simulink model "MBD_If_Action_Subsystem"  (R2021b)
settings: Solver=FixedStepDiscrete  StartTime=0.0  StopTime=10.0  FixedStep=0.001  RelTol=1e-3
libraries: simulink x2
settings Model: Creator=waleed.elshemy  LastModifiedBy=waleed.elshemy
settings OptimizationCC: DefaultParameterBehavior=Inlined  UseDivisionForNetSlopeComputation=on  GainParamInheritBuiltInType=on  UseFloatMulNetSlope=on  InlineInvariantSignals=on  PassReuseOutputArgsAs=Individual arguments  ZeroExternalMemoryAtStartup=off  ZeroInternalMemoryAtStartup=off  NoFixptDivByZeroProtection=on  EfficientFloat2IntCast=on  LifeSpan=1  OptimizeBlockOrder=speed  DifferentSizesBufferReuse=on  EfficientTunableParamExpr=on
settings DebuggingCC: ParameterTunabilityLossMsg=error
settings HardwareCC: ProdLongLongMode=on
settings SFSimCC: MATLABDynamicMemAlloc=off
settings RTWCC: Description=Embedded Coder  SystemTargetFile=ert.tlc  TemplateMakefile=ert_default_tmf
settings CodeAppCC: ForceParamTrailComments=on  IgnoreCustomStorageClasses=off  OperatorAnnotations=on  SimulinkDataObjDesc=on  SFDataObjDesc=on  CustomSymbolStrGlobalVar=rt$N$M  CustomSymbolStrType=$N$M  CustomSymbolStrFcn=$N$M$F  CustomSymbolStrMacro=$N$M  InsertBlockDesc=on
settings ERTTargetCC: TargetLangStandard=C99 (ISO)  GenerateSampleERTMain=on  IncludeMdlTerminateFcn=off  CombineSignalStateStructs=on  SupportComplex=off  SupportContinuousTime=on  InlinedParameterPlacement=NonHierarchical  ERTCustomFileTemplate=example_file_process.tlc  ERTFilePackagingFormat=CompactWithDataFile

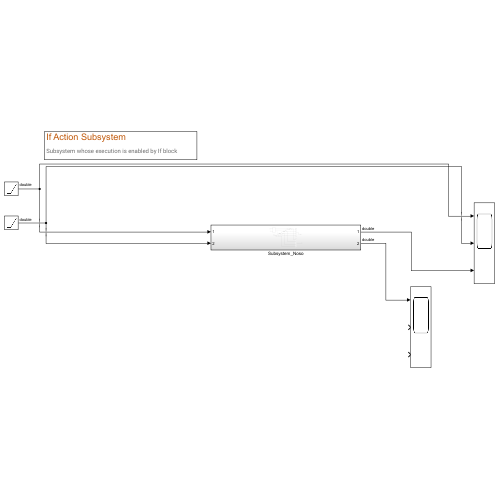
[thumbnail: Simulink's stored preview of the top-level diagram]
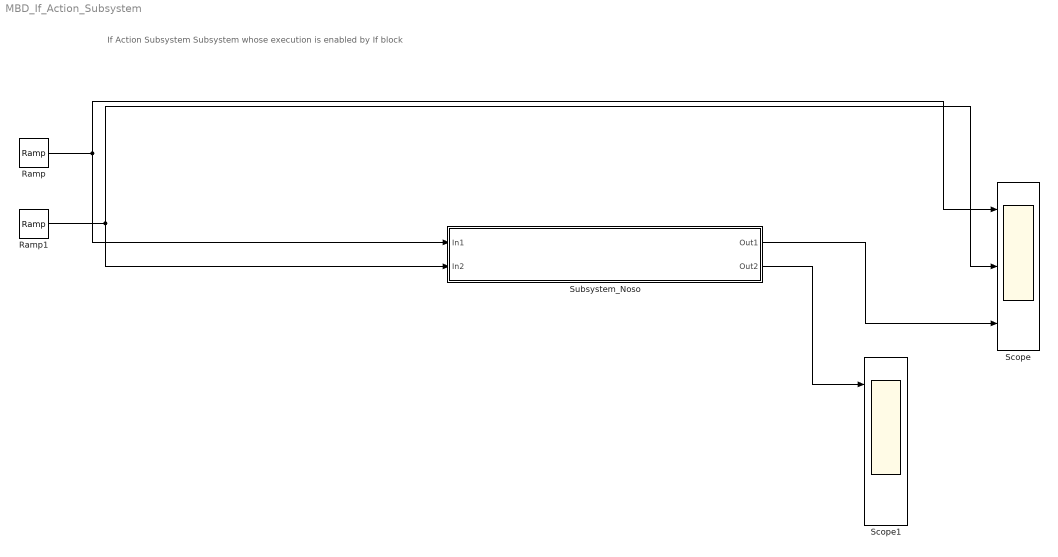
== system MBD_If_Action_Subsystem ==
  note: If Action Subsystem
      | Subsystem whose execution is enabled by If block
  Ramp : simulink/Sources/Ramp  slope=1  start=0  InitialOutput=0
  Ramp1 : simulink/Sources/Ramp  slope=-1  start=0  InitialOutput=10
  Scope : Scope  NumInputPorts=3
  Scope1 : Scope  NumInputPorts=3
  Subsystem_Noso : Subsystem
  wires:
  Ramp/1 -> Subsystem_Noso/1(In1), Scope/1
  Ramp1/1 -> Subsystem_Noso/2(In2), Scope/2
  Subsystem_Noso/1(Out1) -> Scope/3
  Subsystem_Noso/2(Out2) -> Scope1/1

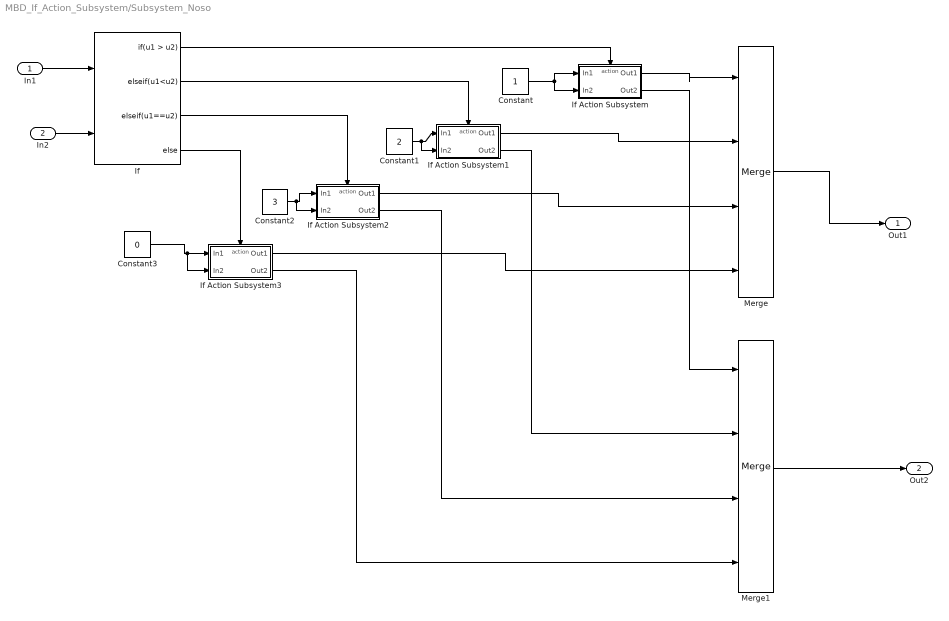
== system MBD_If_Action_Subsystem/Subsystem_Noso ==
  In1 : Inport
  In2 : Inport  Port=2
  Constant : Constant
  Constant1 : Constant  Value=2
  Constant2 : Constant  Value=3
  Constant3 : Constant  Value=0
  If : If  NumInputs=2  IfExpression=u1 > u2  ElseIfExpressions=u1<u2, u1==u2
  If Action Subsystem : Subsystem  TreatAsAtomicUnit=on
  If Action Subsystem1 : Subsystem  TreatAsAtomicUnit=on
  If Action Subsystem2 : Subsystem  TreatAsAtomicUnit=on
  If Action Subsystem3 : Subsystem  TreatAsAtomicUnit=on
  Merge : Merge  Inputs=4
  Merge1 : Merge  Inputs=4
  Out1 : Outport
  Out2 : Outport  Port=2
  wires:
  If/4 -> If Action Subsystem3/Action
  Constant/1 -> If Action Subsystem/1(In1), If Action Subsystem/2(In2)
  Constant2/1 -> If Action Subsystem2/2(In2), If Action Subsystem2/1(In1)
  Constant3/1 -> If Action Subsystem3/2(In2), If Action Subsystem3/1(In1)
  If Action Subsystem3/1(Out1) -> Merge/4
  If Action Subsystem2/1(Out1) -> Merge/3
  If/1 -> If Action Subsystem/Action
  If/2 -> If Action Subsystem1/Action
  Constant1/1 -> If Action Subsystem1/2(In2), If Action Subsystem1/1(In1)
  If Action Subsystem1/1(Out1) -> Merge/2
  In2/1 -> If/2
  Merge/1 -> Out1/1
  If Action Subsystem/1(Out1) -> Merge/1
  If/3 -> If Action Subsystem2/Action
  In1/1 -> If/1
  If Action Subsystem/2(Out2) -> Merge1/1
  If Action Subsystem1/2(Out2) -> Merge1/2
  If Action Subsystem2/2(Out2) -> Merge1/3
  If Action Subsystem3/2(Out2) -> Merge1/4
  Merge1/1 -> Out2/1

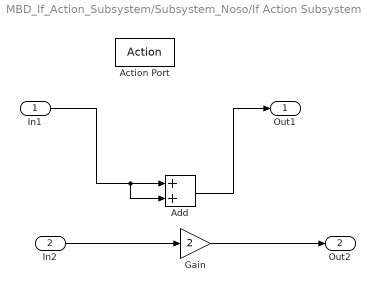
== system MBD_If_Action_Subsystem/Subsystem_Noso/If Action Subsystem ==
  In1 : Inport
  In2 : Inport  Port=2
  Action Port : ActionPort  ActionPortLabel=if(u1 > u2)
  Add : Sum
  Gain : Gain  Gain=2
  Out1 : Outport
  Out2 : Outport  Port=2
  wires:
  In1/1 -> Add/2, Add/1
  Add/1 -> Out1/1
  Gain/1 -> Out2/1
  In2/1 -> Gain/1

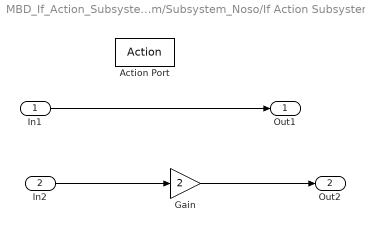
== system MBD_If_Action_Subsystem/Subsystem_Noso/If Action Subsystem1 ==
  In1 : Inport
  In2 : Inport  Port=2
  Action Port : ActionPort  ActionPortLabel=elseif(u1<u2)
  Gain : Gain  Gain=2
  Out1 : Outport
  Out2 : Outport  Port=2
  wires:
  In1/1 -> Out1/1
  Gain/1 -> Out2/1
  In2/1 -> Gain/1

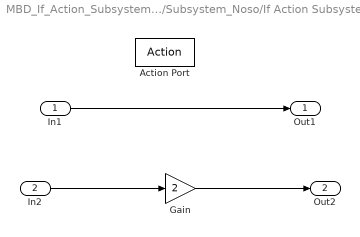
== system MBD_If_Action_Subsystem/Subsystem_Noso/If Action Subsystem2 ==
  In1 : Inport
  In2 : Inport  Port=2
  Action Port : ActionPort  ActionPortLabel=elseif( u1==u2)
  Gain : Gain  Gain=2
  Out1 : Outport
  Out2 : Outport  Port=2
  wires:
  In1/1 -> Out1/1
  Gain/1 -> Out2/1
  In2/1 -> Gain/1

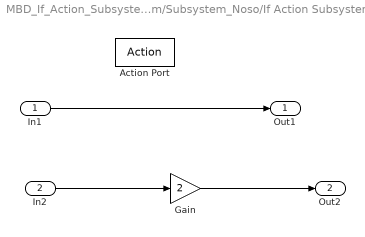
== system MBD_If_Action_Subsystem/Subsystem_Noso/If Action Subsystem3 ==
  In1 : Inport
  In2 : Inport  Port=2
  Action Port : ActionPort  ActionPortLabel=else
  Gain : Gain  Gain=2
  Out1 : Outport
  Out2 : Outport  Port=2
  wires:
  In1/1 -> Out1/1
  Gain/1 -> Out2/1
  In2/1 -> Gain/1
